simulink model "BuckBoost1"  (Simulink 8.0)
settings: Solver=FixedStepDiscrete  StartTime=0.0  StopTime=5  FixedStep=1e-6  RelTol=1e-3
values from neighbouring files (symbols this model uses):
  Imax = 16    [BuckBoost1_Init1.m]
  R = 30    [BuckBoost1_Init1.m]
  Ts = 1e-4    (= 0.0001)    [BuckBoost1_Init1.m]
  Vin = 40    [BuckBoost1_Init1.m]
libraries: powerlib x12, powerlib_extras x2
settings Model: Creator=zxn  LastModifiedBy=Harri
settings DataIOCC: SignalLoggingSaveFormat=ModelDataLogs
settings DebuggingCC: FcnCallInpInsideContextMsg=UseLocalSettings
settings GRTTargetCC: CombineOutputUpdateFcns=off  GRTInterface=on

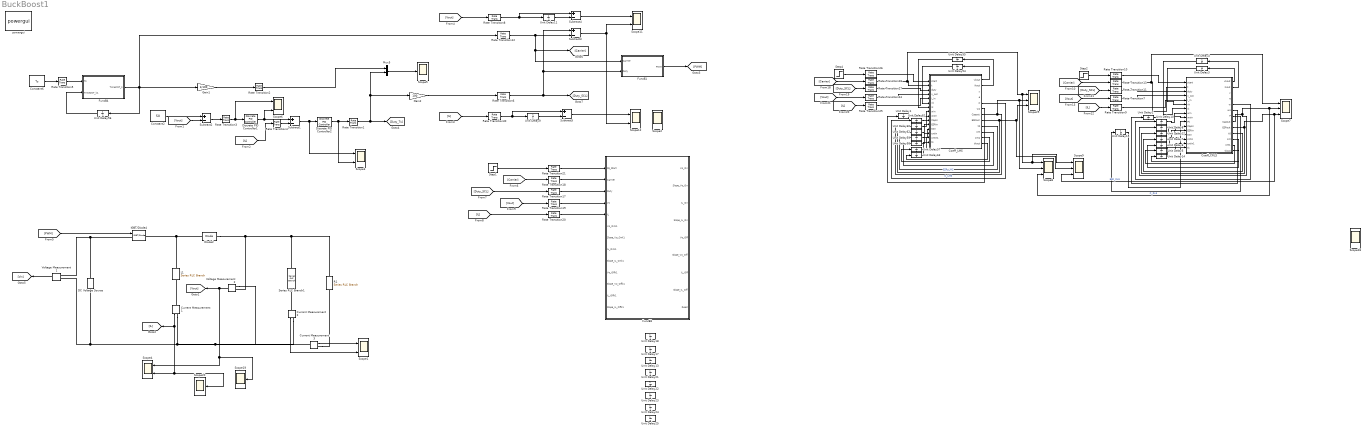
== system BuckBoost1 ==
  Coeff_CRLS : MATLAB Function  TreatAsAtomicUnit=on
  Coeff_LMS : MATLAB Function  TreatAsAtomicUnit=on
  Constant2 : Constant  Value=50
  Constant6 : Constant  Value=Ts
  Current Measurement1 : powerlib/Measurements/Current Measurement  PhasorSimulation=off  OutputType=Complex  PSBequivalent=0
  Current Measurement2 : powerlib/Measurements/Current Measurement  PhasorSimulation=off  OutputType=Complex  PSBequivalent=0
  Current Measurement3 : powerlib/Measurements/Current Measurement  PhasorSimulation=off  OutputType=Complex  PSBequivalent=0
  DC Voltage Source : powerlib/Electrical Sources/DC Voltage Source  Amplitude=Vin  Measurements=None
  Diode2 : powerlib/Power Electronics/Diode  Ron=0.001  Lon=0  Vf=0.8  IC=0  UseSnubber=off  Rs=inf  Cs=inf  Measurements=off
  Discrete PID Controller1 : powerlib_extras/Discrete  Control Blocks/Discrete PID Controller  Kp=1.4  Ki=0.4  Kd=0  TcD=0  Par_Limits=[1 -1]*Imax  Init=0  Ts=Ts
  Discrete PID Controller2 : powerlib_extras/Discrete  Control Blocks/Discrete PID Controller  Kp=30e-3  Ki=50e-3  Kd=0  TcD=0  Par_Limits=[1 -1]*0.9  Init=0  Ts=Ts
  FuncB1 : MATLAB Function  TreatAsAtomicUnit=on
  FuncB3 : MATLAB Function  TreatAsAtomicUnit=on
  FuncB4 : MATLAB Function  TreatAsAtomicUnit=on
  Gain1 : Gain  Gain=1/100
  Gain2 : Gain  Gain=100
  IGBT/Diode4 : powerlib/Power Electronics/IGBT//Diode  Ron=1e-3  Rs=1e5  Cs=inf  Measurements=off
  L1 : powerlib/Elements/Series RLC Branch  LConnTagsString=__new0  RConnTagsString=__new0  BranchType=L  Resistance=1  Inductance=5e-3  SetiL0=off  InitialCurrent=0  Capacitance=1e-6  Setx0=off  InitialVoltage=0  Measurements=None
  Mux5 : Mux  Inputs=2
  R1 : powerlib/Elements/Series RLC Branch  LConnTagsString=__new0  RConnTagsString=__new0  BranchType=R  Resistance=R  Inductance=1e-3  SetiL0=off  InitialCurrent=0  Capacitance=1e-6  Setx0=off  InitialVoltage=0  Measurements=None
  Rate Transition{1..2,6..13,17..21,24..28,30} (21 alike) : RateTransition  OutPortSampleTime=1e-6
  Rate Transition3 : RateTransition  OutPortSampleTime=Ts
  Rate Transition4 : RateTransition  OutPortSampleTime=Ts
  Rate Transition5 : RateTransition  X0=Ts  OutPortSampleTime=1e-6
  Scope{1,3..4,6,11..12,28} (7 alike) : Scope  NumInputPorts=2
      Scope1 settings: TickLabels=on  TimeRange=10  YMin=210~0  YMax=320~47.5  SaveName=var1
      Scope11 settings: TickLabels=on  TimeRange=5  YMin=-0.06~-40  YMax=0.07~65  SaveName=var10  MaxDataPoints=1000000
      Scope12 settings: TickLabels=on  TimeRange=5  YMin=-0.011~-40  YMax=0.01~65  SaveName=var13  MaxDataPoints=1000000
      Scope28 settings: TickLabels=on  TimeRange=5  YMin=0~0  YMax=350000~325000  SaveName=var25  MaxDataPoints=1000000
      Scope3 settings: TickLabels=on  TimeRange=1.5  YMin=0.5~0  YMax=0.605~1  SaveName=var4
      Scope4 settings: TickLabels=on  YMin=41.5~2.4  YMax=50~4.3  SaveName=var
      Scope6 settings: TickLabels=on  TimeRange=1.5  YMin=0.5~0  YMax=0.605~1  SaveName=var2
  Scope19 : Scope
      settings: TickLabels=on  YMin=41.5  YMax=50  SaveName=Vout
  Scope2 : Scope  NumInputPorts=4
      settings: TickLabels=on  TimeRange=5  YMin=-0.011~-40~-5~-5  YMax=0.01~65~5~5  SaveName=var3  MaxDataPoints=1000000
  Scope20 : Scope
      settings: TickLabels=on  YMin=41.5  YMax=50  SaveName=Iin
  Scope{7..9,29} (4 alike) : Scope  NumInputPorts=3
      Scope29 settings: TickLabels=on  TimeRange=5  YMin=0~-0.0001~0  YMax=100~0.0013~0.12  SaveName=var26  MaxDataPoints=1000000
      Scope7 settings: TickLabels=on  TimeRange=5  YMin=0~-3.75e-06~-175  YMax=100~0~0  SaveName=var6  MaxDataPoints=1000000
      Scope8 settings: TickLabels=on  TimeRange=5  YMin=0~-0.0001~-0.0075  YMax=100~0.0013~0.0325  SaveName=var7  MaxDataPoints=1000000
      Scope9 settings: TickLabels=on  TimeRange=5  YMin=0~-175~0  YMax=100~25~0.12  SaveName=var8  MaxDataPoints=1000000
  Scope5 : Scope
      settings: TickLabels=on  TimeRange=1.5  YMin=0.5  YMax=0.605  SaveName=var5  MaxDataPoints=100000
  Series RLC Branch1 : powerlib/Elements/Series RLC Branch  LConnTagsString=__new0  RConnTagsString=__new0  BranchType=RC  Resistance=75e-3*1  Inductance=1e-3  SetiL0=off  InitialCurrent=0  Capacitance=1e-3*1.25  Setx0=off  InitialVoltage=500  Measurements=None
  Step1 : Step  Time=3.3  SampleTime=0
  Step2 : Step  Time=3.3  SampleTime=0
  Step4 : Step  Time=3.3  SampleTime=0
  Subtract1 : Sum  Inputs=+-  SampleTime=Ts
  Subtract{2..5} (4 alike) : Sum  Inputs=+-
  Unit Delay{1..14,17..18,21..25,54..63} (31 alike) : UnitDelay  SampleTime=1e-6
  Unit Delay15 : UnitDelay  InitialCondition=100  SampleTime=1e-6
  Voltage Measurement1 : powerlib/Measurements/Voltage Measurement  PhasorSimulation=off  OutputType=Complex  PSBequivalent=0
  Voltage Measurement2 : powerlib/Measurements/Voltage Measurement  PhasorSimulation=off  OutputType=Complex  PSBequivalent=0
  powergui : powerlib/powergui  Priority=2  SimulationMode=Discrete  SolverType=Tustin  SampleTime=1e-6  frequency=60  SPID=off  DisableSnubberDevices=off  DisableRonSwitches=off  DisableVfSwitches=off  SwTol=0  Interpol=off  DisplayEquations=off  FunctionMessages=off  frequencyindice=0  Pbase=100e6  ErrMax=1e-4  Iterations=50  UnitsV=kV  UnitsW=MW  echomessages=off  HookPort=off  EnableUseOfTLC=off  x0status=blocks  RestoreLinks=warning  ResistiveCurrentMeasurement=off  Frange=[0:2:500]  Ylog=off  Xlog=off  ShowGrid=off  save=off  variable=ZData  structure=ScopeData  ZoomFFT=on  StartTime=0.0  cycles=1  DisplayStyle=1  fundamental=60  FreqAxis=off  MaxFrequency=8000  frequencyindicesteady=1  RmsSteady=1  display=off  Ts=0  methode=off
  wires:
  Constant2/1 -> Subtract2/1
  Subtract2/1 -> Rate Transition3/1
  Voltage Measurement2/1 -> Scope19/1, Scope4/1, [Vout]
  Current Measurement1/1 -> [IL], Scope20/1, Scope4/2
  Current Measurement3/1 -> Scope1/1
  Current Measurement2/1 -> Scope1/2
  Rate Transition2/1 -> Mux5/1
  Rate Transition3/1 -> Discrete PID Controller1/1, Scope6/1
  Discrete PID Controller1/1 -> Subtract1/1, Scope6/2
  Subtract1/1 -> Discrete PID Controller2/1, Scope3/1
  Rate Transition4/1 -> Subtract1/2
  [IL] -> Rate Transition4/1
  [Vout] -> Subtract2/2
  Discrete PID Controller2/1 -> Rate Transition1/1, Scope3/2
  Rate Transition1/1 -> Mux5/2, Gain2/1, [Duty_Ts]
  Mux5/1 -> Scope5/1
  Rate Transition6/1 -> [Duty_SCL], Subtract3/1, FuncB1/2(Duty)
  Rate Transition8/1 -> Unit Delay11/1, Subtract4/1
  [PWM] -> IGBT/Diode4/1
  Voltage Measurement1/1 -> [Vin]
  Rate Transition5/1 -> FuncB4/1(Ts)
  Constant6/1 -> Rate Transition5/1
  Unit Delay56/1 -> FuncB4/2(TimeCNT_k1)
  FuncB4/1(TimeCNT_k) -> Unit Delay56/1, Gain1/1, Rate Transition12/1
  Gain1/1 -> Rate Transition2/1
  Gain2/1 -> Rate Transition6/1
  Subtract3/1 -> Scope11/2, Scope12/2
  Rate Transition12/1 -> Subtract3/2, [Carrier], FuncB1/1(Carrier)
  Unit Delay11/1 -> Subtract4/2
  Subtract4/1 -> Scope11/1
  [Vout] -> Rate Transition8/1
  [Carrier] -> Rate Transition18/1
  [Duty_SCL] -> Rate Transition17/1
  Step1/1 -> Rate Transition21/1
  [IL] -> Rate Transition20/1
  [Vout] -> Rate Transition19/1
  FuncB1/1(PWM) -> [PWM]
  Rate Transition21/1 -> FuncB3/1(SS_Start)
  Rate Transition18/1 -> FuncB3/2(Carrier)
  Rate Transition17/1 -> FuncB3/3(Duty)
  Rate Transition19/1 -> FuncB3/4(Vc)
  Rate Transition20/1 -> FuncB3/5(IL)
  [IL] -> Rate Transition30/1
  Unit Delay9/1 -> Subtract5/2
  Rate Transition30/1 -> Unit Delay9/1, Subtract5/1
  Subtract5/1 -> Scope12/1
  Coeff_LMS/1(vkout) -> Unit Delay54/1
  Unit Delay54/1 -> Coeff_LMS/6(vk)
  Coeff_LMS/2(ikout) -> Unit Delay55/1
  Unit Delay55/1 -> Coeff_LMS/7(ik)
  Unit Delay61/1 -> Coeff_LMS/8(win)
  Unit Delay60/1 -> Coeff_LMS/10(Capin)
  Unit Delay59/1 -> Coeff_LMS/12(t0in)
  Unit Delay58/1 -> Coeff_LMS/13(cntin)
  Unit Delay57/1 -> Coeff_LMS/14(cntin1)
  Coeff_LMS/11(cnt1) -> Unit Delay57/1
  Coeff_LMS/10(cnt) -> Unit Delay58/1
  Coeff_LMS/9(t0) -> Unit Delay59/1
  Coeff_LMS/7(Capout) -> Scope8/2, Scope29/2, Unit Delay60/1  "C_LMS"
  Coeff_LMS/5(w) -> Unit Delay61/1
  [Carrier] -> Rate Transition28/1
  [Duty_SCL] -> Rate Transition27/1
  Step4/1 -> Rate Transition26/1
  [Vout] -> Rate Transition24/1
  [IL] -> Rate Transition25/1
  Rate Transition25/1 -> Coeff_LMS/5(i_in)
  Rate Transition24/1 -> Coeff_LMS/4(v_out)
  Rate Transition27/1 -> Coeff_LMS/3(duty)
  Rate Transition28/1 -> Scope9/1, Scope8/1, Scope29/1, Coeff_LMS/2(t)
  Rate Transition26/1 -> Coeff_LMS/1(start)
  Unit Delay62/1 -> Coeff_LMS/11(ESRin)
  Coeff_LMS/8(ESRout) -> Scope9/2, Scope29/3, Unit Delay62/1  "ESR_LMS"
  Unit Delay63/1 -> Coeff_LMS/15(tk)
  Coeff_LMS/12(tkout) -> Unit Delay63/1
  Unit Delay1/1 -> Coeff_LMS/9(woin)
  Coeff_LMS/6(wo) -> Unit Delay1/1
  Coeff_CRLS/1(vkout) -> Unit Delay3/1
  Unit Delay3/1 -> Coeff_CRLS/6(vk)
  Coeff_CRLS/2(ikout) -> Unit Delay4/1
  Unit Delay4/1 -> Coeff_CRLS/7(ik)
  Unit Delay10/1 -> Coeff_CRLS/8(win)
  Unit Delay8/1 -> Coeff_CRLS/11(Capin)
  Unit Delay7/1 -> Coeff_CRLS/13(t0in)
  Unit Delay6/1 -> Coeff_CRLS/14(cntin)
  Unit Delay5/1 -> Coeff_CRLS/15(cntin1)
  Coeff_CRLS/12(cnt1) -> Unit Delay5/1
  Coeff_CRLS/11(cnt) -> Unit Delay6/1
  Coeff_CRLS/10(t0) -> Unit Delay7/1
  Coeff_CRLS/8(Capout) -> Unit Delay8/1, Scope8/3, Scope7/2  "C_RLS"
  Coeff_CRLS/5(w) -> Unit Delay10/1
  [Carrier] -> Rate Transition13/1
  [Duty_SCL] -> Rate Transition11/1
  Step2/1 -> Rate Transition10/1
  [Vout] -> Rate Transition7/1
  [IL] -> Rate Transition9/1
  Rate Transition9/1 -> Coeff_CRLS/5(i_in)
  Rate Transition7/1 -> Coeff_CRLS/4(v_out)
  Rate Transition11/1 -> Coeff_CRLS/3(duty)
  Rate Transition13/1 -> Scope7/1, Coeff_CRLS/2(t)
  Rate Transition10/1 -> Coeff_CRLS/1(start)
  Unit Delay12/1 -> Coeff_CRLS/12(ESRin)
  Coeff_CRLS/9(ESRout) -> Scope9/3, Scope7/3, Unit Delay12/1  "ESR_RLS"
  Unit Delay14/1 -> Coeff_CRLS/16(tk)
  Coeff_CRLS/13(tkout) -> Unit Delay14/1
  Unit Delay2/1 -> Coeff_CRLS/9(woin)
  Coeff_CRLS/6(wo) -> Unit Delay2/1
  Unit Delay15/1 -> Coeff_CRLS/10(Pk)
  Coeff_CRLS/7(P) -> Unit Delay15/1
  connections:
  DC Voltage Source/RConn1 -- IGBT/Diode4/LConn1 -- Voltage Measurement1/LConn1
  Diode2/RConn1 -- IGBT/Diode4/RConn1 -- L1/RConn1
  Current Measurement3/LConn1 -- Current Measurement2/RConn1 -- Voltage Measurement2/LConn1 -- Current Measurement1/RConn1 -- DC Voltage Source/LConn1 -- Voltage Measurement1/LConn2
  Current Measurement1/LConn1 -- L1/LConn1
  Diode2/LConn1 -- R1/RConn1 -- Series RLC Branch1/RConn1 -- Voltage Measurement2/LConn2
  Current Measurement2/LConn1 -- Series RLC Branch1/LConn1
  Current Measurement3/RConn1 -- R1/LConn1

== matlab function Coeff_CRLS ==
  data: vkout output double; ikout output double; start input double; t input double; duty input double; v_out input double; i_in input double; vk input double; ik input double; win input double; woin input double; Pk input double; Capin input double; ESRin input double; y output double; e output double; w output double; wo output double; P output double; Capout output double; ESRout output double; t0in input double; t0 output double; cntin input double; cnt output double; cntin1 input double; cnt1 output double; tk input double; tkout output double
function [vkout, ikout, y, e, w, wo, P, Capout, ESRout, t0, ...
    cnt, cnt1, tkout]  = ...
    Coeff_CRLS_Est(start,t,duty,v_out,i_in, vk, ik, ...
    win, woin, Pk, Capin, ESRin, t0in, ...
    cntin, cntin1, tk)
%#codegen

% *** Time Partition ******************************************************
sampling_time = 1e-6;

offset = t - duty;

OFFSET_ON_START_abs = 0+5; % for t
OFFSET_ON_END_rel = -5; % for offset
OFFSET_OFF_START_rel = 5; % for offset
OFFSET_OFF_END_abs = 90+5; % for t
% --- end of Time Partition -----------------------------------------------

% *** Init ****************************************************************
lambda = 0.01;%0.05;%0.2;%0.995;%0.9;%0.6;
% delta = 1/100; % NOTE: put this value in delay unit of P
% RECORDED GOOD: lambda = 0.1; Pk init = 100
% <<~~~ uON(t) = w0 + w1*t ~~~~~~~~~~~~~~~~~~~~~~~~~~~~~~~~~~~~~~~~~~~~~~>>

% ... estimator output ...
y = 0.0;
e = 0.0;

% ... inputs ...

% ... coefficients ...
w = win;
wo = woin;

% ... algorithm specific tools ...
P = Pk;

% --- end of Init ---------------------------------------------------------

% *** Misc. ***************************************************************

Capout = Capin;
ESRout = ESRin;
t0 = t0in;
tkout = tk;
vkout = vk;
ikout = ik;

%noiseAmp = 0.1;

% --- end of Misc. --------------------------------------------------------


cnt = cntin; cnt1 = cntin1;

% *** sampling occure at **************************************************
SAMPLE_1t_abs = OFFSET_ON_START_abs+10;
SAMPLE_2t_rel = OFFSET_ON_END_rel-10;
SAMPLE_3t_rel = OFFSET_OFF_START_rel+10;
SAMPLE_4t_abs = OFFSET_OFF_END_abs-10;
% --- end of sampling occure at -------------------------------------------

if(start==1)
    % *** State: ON *******************************************************
    if(t > OFFSET_ON_START_abs && offset < OFFSET_ON_END_rel)
        % estimate the "C"
        %if(t > OFFSET_ON_START_abs && t<= OFFSET_ON_START_abs+1)% ---> +2)
        %    t0 = t;
        %    cnt = 0; %need
        %else%end% --> else
        if (t < t0)
            cnt = 0;
        end
        
        if ( t > SAMPLE_1t_abs && t<=SAMPLE_1t_abs+2)
            cnt = cntin + 1;
            
            vkout = v_out;
            tkout = t;
        elseif ( offset > SAMPLE_2t_rel && offset <= SAMPLE_2t_rel+2)
            cnt = cntin + 1;
            
            del_v = v_out - vk;
            del_t = (t - tk) * sampling_time;
            slope_v = del_v / del_t;
            
            d = slope_v; % this is "y"            
            u = v_out; % this is "x"
            
            % now CRLS for the only "w"
            kden = lambda + u*P*u;
            knom = P*u;
            k = knom/kden;
            
            y = w * u;
            e = d - y;
            
            w = w + k*e;
            
            P = (P - k*u*P)/lambda;
                
        end
        
    end
    if(offset >= OFFSET_ON_END_rel && offset <= OFFSET_ON_END_rel+1)
        %Capout = -w0/w1/30;%*sampling_time;%R=30
        Capout = -1/30/win;
    end
    % --- end State: ON ---------------------------------------------------
    
    % *** State: OFF ******************************************************
    if(offset > OFFSET_OFF_START_rel && t < OFFSET_OFF_END_abs) % OFF
        % estimate the "ESR"
        
        if (t < t0)
            cnt = 0;
        end
        
        if ( offset > SAMPLE_3t_rel && offset<=SAMPLE_3t_rel+2)
            cnt = cntin + 1;
            
            vkout = v_out;
            ikout = i_in;
            tkout = t;
        elseif ( t > SAMPLE_4t_abs && t <= SAMPLE_4t_abs+2)
            cnt = cntin + 1;
            
            del_v = v_out - vk;
            del_i = i_in - ik;
            del_t = (t - tk) * sampling_time;
            slope_v = del_v / del_t;
            slope_i = del_i / del_t;
            
            d = slope_v - (i_in - v_out/30)/Capin; % this is "y"            
            u = slope_i - slope_v/30; % this is "x"
            
            % now LMS for the only "w"
            kden = lambda + u*P*u;
            knom = P*u;
            k = knom/kden;
            
            y = wo * u;
            e = d - y;
            
            wo = wo + k*e;
            
            P = (P - k*u*P)/lambda;
                
        end
        
    end
    if(t >= OFFSET_OFF_END_abs && t <= OFFSET_OFF_END_abs+1)
        ESRout = wo;
    end
    % --- end State: OFF --------------------------------------------------

    % -----------------
end

== matlab function FuncB3 ==
  data: SS_Start input double; Carrier input double; Duty input double; Vc input double; IL input double; Vo_Onk1 input double; Slope_Vo_Onk1 input double; IL_Onk1 input double; Slope_IL_Onk1 input double; Vo_Offk1 input double; Slope_Vo_Offk1 input double; IL_Offk1 input double; Vo_On output double; Slope_Vo_On output double; IL_On output double; Slope_IL_On output double; Vo_Off output double; Slope_Vo_Off output double; IL_Off output double; Slope_IL_Off output double; Read output double; Slope_IL_Offk1 input double
function [Vo_On,Slope_Vo_On,IL_On,Slope_IL_On,Vo_Off,Slope_Vo_Off,IL_Off,Slope_IL_Off,Read] = Sample(SS_Start,Carrier,Duty,Vc,IL,Vo_Onk1,Slope_Vo_Onk1,IL_Onk1,Slope_IL_Onk1,Vo_Offk1,Slope_Vo_Offk1,IL_Offk1,Slope_IL_Offk1)

Err1=(Carrier - Duty);  Tsimulation=1e-6;%1e-6;
%DtT_On=Duty*Tsimulation;    DtT_Off=(100 - Duty)*Tsimulation;%%!! 100 should be repaced Correspondingly by CNT_Max
Fix10us=10e-6;
if(SS_Start==1)
    if(Err1>=-12)&&(Err1<-11) %%Just After Switch-On; (Err1>=-2)&&(Err1<-1); (Carrier==3)
        Vo_On=Vc; IL_On=IL;
        Read=0;
        Slope_Vo_On=Slope_Vo_Onk1; Slope_IL_On=Slope_IL_Onk1;
        Slope_Vo_Off=Slope_Vo_Offk1; Slope_IL_Off=Slope_IL_Offk1;
        Vo_Off=Vo_Offk1; IL_Off=IL_Offk1;
    elseif((Err1>=-2)&&(Err1<-1)) %%Next moment Switch-Off
        %Slope_Vo_On=(Vc - Vo_Onk1)/DtT_On; Slope_IL_On=(IL - IL_Onk1)/DtT_On;
        Slope_Vo_On=(Vc - Vo_Onk1)/Fix10us; Slope_IL_On=(IL - IL_Onk1)/Fix10us;
        Vo_On=Vo_Onk1; IL_On=IL_Onk1;
        Slope_Vo_Off=Slope_Vo_Offk1; Slope_IL_Off=Slope_IL_Offk1; Read=0; 
        Vo_Off=Vo_Offk1; IL_Off=IL_Offk1;
    elseif(Carrier==89) %%Just After Switch Off; Carrier==98; (Err1>3)&&(Err1<=4)
        Vo_Off=Vc;  IL_Off=IL;
        Slope_Vo_Off=Slope_Vo_Offk1;  Slope_IL_Off=Slope_IL_Offk1;
        Slope_Vo_On=Slope_Vo_Onk1;  Slope_IL_On=Slope_IL_Onk1; Read=0;
        Vo_On=Vo_Onk1; IL_On=IL_Onk1;
    elseif(Carrier==99) %%Next moment Switch-On
        %Slope_Vo_Off=(Vc - Vo_Offk1)/DtT_Off;  Slope_IL_Off=(IL - IL_Offk1)/DtT_Off;
        Slope_Vo_Off=(Vc - Vo_Offk1)/Fix10us;  Slope_IL_Off=(IL - IL_Offk1)/Fix10us;
        Vo_Off=Vo_Offk1;  IL_Off=IL_Offk1;
        Read=1;
        Slope_Vo_On=Slope_Vo_Onk1; Slope_IL_On=Slope_IL_Onk1;
        Vo_On=Vo_Onk1; IL_On=IL_Onk1;
    else
        Vo_On=Vo_Onk1; Slope_Vo_On=Slope_Vo_Onk1; IL_On=IL_Onk1; Slope_IL_On=Slope_IL_Onk1; %%On_Readk1
        Vo_Off=Vo_Offk1;  Slope_Vo_Off=Slope_Vo_Offk1;  IL_Off=IL_Offk1;  Slope_IL_Off=Slope_IL_Offk1; Read=0; %%Off_Readk1
    end
else
    Vo_On=49;  Slope_Vo_On=0.5;  IL_On=4;  Slope_IL_On=0.2;
    Vo_Off=50;  Slope_Vo_Off=0.5;  IL_Off=3.8;  Slope_IL_Off=0.2; Read=0;
end

end

== matlab function Coeff_LMS ==
  data: vkout output double; ikout output double; start input double; t input double; duty input double; v_out input double; i_in input double; vk input double; ik input double; win input double; woin input double; Capin input double; ESRin input double; y output double; e output double; w output double; wo output double; Capout output double; ESRout output double; t0in input double; t0 output double; cntin input double; cnt output double; cntin1 input double; cnt1 output double; tk input double; tkout output double
function [vkout, ikout, y, e, w, wo, Capout, ESRout, t0, ...
    cnt, cnt1, tkout]  = ...
    Coeff_LMS_Est(start,t,duty,v_out,i_in, vk, ik, ...
    win, woin, Capin, ESRin, t0in, ...
    cntin, cntin1, tk)
%#codegen

% *** Time Partition ******************************************************
sampling_time = 1e-6;

offset = t - duty;

OFFSET_ON_START_abs = 0+5; % for t
OFFSET_ON_END_rel = -5; % for offset
OFFSET_OFF_START_rel = 5; % for offset
OFFSET_OFF_END_abs = 90+5; % for t
% --- end of Time Partition -----------------------------------------------

% *** Init ****************************************************************
beta = 0.5;

% <<~~~ uON(t) = w0 + w1*t ~~~~~~~~~~~~~~~~~~~~~~~~~~~~~~~~~~~~~~~~~~~~~~>>

% ... estimator output ...
y = 0.0;
e = 0.0;

% ... inputs ...

% ... coefficients ...
w = win;
wo = woin;

% ... algorithm specific tools ...


% --- end of Init ---------------------------------------------------------

% *** Misc. ***************************************************************

Capout = Capin;
ESRout = ESRin;
t0 = t0in;
tkout = tk;
vkout = vk;
ikout = ik;

%noiseAmp = 0.1;

% --- end of Misc. --------------------------------------------------------


cnt = cntin; cnt1 = cntin1;

% *** sampling occure at **************************************************
SAMPLE_1t_abs = OFFSET_ON_START_abs+10;
SAMPLE_2t_rel = OFFSET_ON_END_rel-10;
SAMPLE_3t_rel = OFFSET_OFF_START_rel+10;
SAMPLE_4t_abs = OFFSET_OFF_END_abs-10;
% --- end of sampling occure at -------------------------------------------

if(start==1)
    % *** State: ON *******************************************************
    if(t > OFFSET_ON_START_abs && offset < OFFSET_ON_END_rel)
        % estimate the "C"
        %if(t > OFFSET_ON_START_abs && t<= OFFSET_ON_START_abs+1)% ---> +2)
        %    t0 = t;
        %    cnt = 0; %need
        %else%end% --> else
        if (t < t0)
            cnt = 0;
        end
        
        if ( t > SAMPLE_1t_abs && t<=SAMPLE_1t_abs+2)
            cnt = cntin + 1;
            
            vkout = v_out;
            tkout = t;
        elseif ( offset > SAMPLE_2t_rel && offset <= SAMPLE_2t_rel+2)
            cnt = cntin + 1;
            
            del_v = v_out - vk;
            del_t = (t - tk) * sampling_time;
            slope_v = del_v / del_t;
            
            d = slope_v; % this is "y"            
            u = v_out; % this is "x"
            
            % now LMS for the only "w"
            rms = (u*u)/2;
            y = w * u;
            e = d - y;
            
            w = w + beta*e*u/rms;
                
        end
        
    end
    if(offset >= OFFSET_ON_END_rel && offset <= OFFSET_ON_END_rel+1)
        %Capout = -w0/w1/30;%*sampling_time;%R=30
        Capout = -1/30/win;
    end
    % --- end State: ON ---------------------------------------------------
    
    % *** State: OFF ******************************************************
    if(offset > OFFSET_OFF_START_rel && t < OFFSET_OFF_END_abs) % OFF
        % estimate the "ESR"
        
        if (t < t0)
            cnt = 0;
        end
        
        if ( offset > SAMPLE_3t_rel && offset<=SAMPLE_3t_rel+2)
            cnt = cntin + 1;
            
            vkout = v_out;
            ikout = i_in;
            tkout = t;
        elseif ( t > SAMPLE_4t_abs && t <= SAMPLE_4t_abs+2)
            cnt = cntin + 1;
            
            del_v = v_out - vk;
            del_i = i_in - ik;
            del_t = (t - tk) * sampling_time;
            slope_v = del_v / del_t;
            slope_i = del_i / del_t;
            
            d = slope_v - (i_in - v_out/30)/Capin; % this is "y"            
            u = slope_i - slope_v/30; % this is "x"
            
            % now LMS for the only "w"
            rms = (u*u)/2;
            y = wo * u;
            e = d - y;
            
            wo = wo + beta*e*u/rms;
                
        end
        
    end
    if(t >= OFFSET_OFF_END_abs && t <= OFFSET_OFF_END_abs+1)
        ESRout = wo;
    end
    % --- end State: OFF --------------------------------------------------

    % -----------------
end

== matlab function FuncB1 ==
  data: PWM output double; Carrier input double; Duty input double
function PWM  = Sample(Carrier,Duty)

Err1=(Duty - Carrier);
%%Single Switch PWM Signal Generation!
if(Err1>0)
    PWM=1;
else
    PWM=0;
end

end

== matlab function FuncB4 ==
  data: Ts input double; TimeCNT_k1 input double; TimeCNT_k output double
function TimeCNT_k  = IabSlope(Ts,TimeCNT_k1)

Tsimulation=1e-6;%1e-6;
CNT_Ts=Ts/Tsimulation - 1; %%100
%%Vap,Vbt Calculation
if(TimeCNT_k1>=CNT_Ts)
    TimeCNT_k=0;
else
    TimeCNT_k=TimeCNT_k1 + 1;
end

end
